simulink model "BatteryCCCV"  (R2023b)
settings: Solver=VariableStepAuto  StartTime=0.0  StopTime=5*23*3600  FixedStep=Ts  RelTol=1e-3  EnableMultiTasking=on
PreLoadFcn:
  | BatteryCCCVData;
values from neighbouring files (symbols this model uses):
  Ki = 10    [PVSystem_data.m]    (also in Simulink_INPUT_DATA_modified.m)
  Kp = 100    [PVSystem_data.m]    (also in Simulink_INPUT_DATA_modified.m)
  sim_avg_effectiveness_factor = mean(effectiveness_factors)    [Simulink_INPUT_DATA_modified.m]
  sim_general_loss_factor = general_loss_factor    [Simulink_INPUT_DATA_modified.m]
  sim_soiling_loss_factor = soiling_loss_factor    [Simulink_INPUT_DATA_modified.m]
  Ts = 1    [PVSystem_data.m]    (also in Simulink_INPUT_DATA_modified.m)
libraries: nesl_utility x4, fl_lib x3, simulink x2, batteryecm_lib x1, BatteryCurrentManagement x1
CloseFcn:
  | try
  |     close(h1_BatteryCCCV)
  | catch
  | end
  | 
  | clear h1_BatteryCCCV
  | 
  | clear BatteryCCCVSimlog
  | clear BatteryCCCVLogsout
  | 
  | clear AH SOC_vec T_vec R0_mat R1_mat tau1_mat
  | clear V0_mat initialSOC Ts vMax Kp Ki Kaw
  | clear cell_area h_conv thermal_mass
Description:
  | Battery charging and discharging
settings Model: Creator=The MathWorks, Inc.  LastModifiedBy=z004p7rb
settings SolverCC: AlgebraicLoopSolver=TrustRegion  MaxZcPerStep=1
settings DataIOCC: MaxDataPoints=370000  ReturnWorkspaceOutputs=off  SignalLoggingName=BatteryCCCVLogsout
settings OptimizationCC: ReuseModelBlockBuffer=off  LifeSpan=inf
settings DebuggingCC: UnconnectedInputMsg=warning  UnconnectedOutputMsg=warning  UnconnectedLineMsg=warning  SFUnexpectedBacktrackingDiag=warning  SFNoUnconditionalDefaultTransitionDiag=warning  SFExecutionAtInitializationDiag=none  ArithmeticOperatorsInVariantConditions=warning
settings ModelReferenceCC: EnableRefExpFcnMdlSchedulingChecks=on
settings SFSimCC: SimUseLocalCustomCode=off  CustomCodeUndefinedFunction=UseInterfaceOnly
settings RTWCC: RTWUseLocalCustomCode=off  DLArmComputeVersion=19.05
settings CodeAppCC: StateflowObjectComments=on
settings GRTTargetCC: TargetLangStandard=C89/C90 (ANSI)
settings ConfigComp: CovMetricSettings=dw  CovSaveCumulativeToWorkspaceVar=on  CovSaveSingleToWorkspaceVar=on  CovExternalEMLEnable=off
settings SimscapeCC: SimscapeLogType=all  SimscapeLogSimulationStatistics=on  SimscapeLogName=BatteryCCCVSimlog  SimscapeLogLimitData=off  SimscapeLogDataHistory=370000

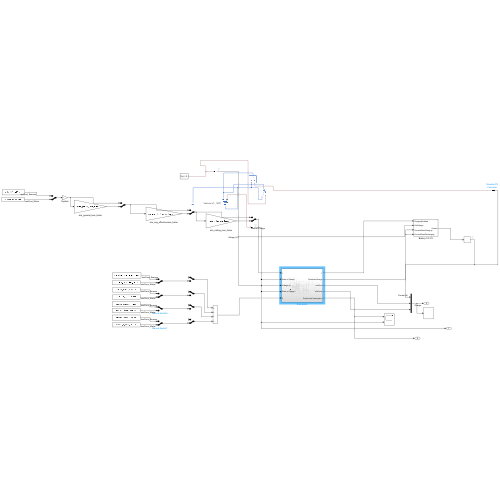
[thumbnail: Simulink's stored preview of the top-level diagram]
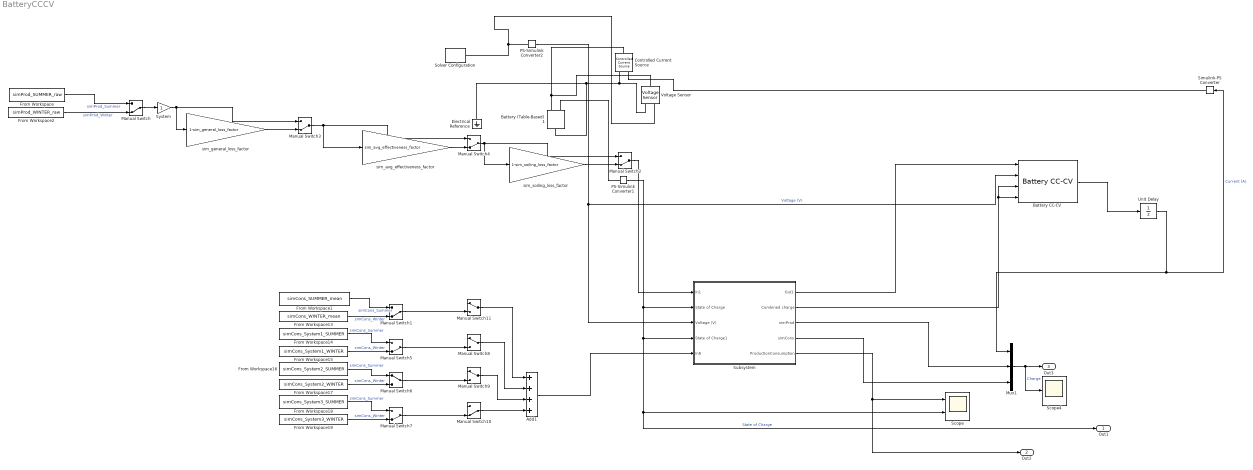
== system BatteryCCCV ==
  Add1 : Sum  Inputs=++++
  Battery (Table-Based)1 : batteryecm_lib/Battery (Table-Based)  Tag={'toolbox/physmod/battery/shared_library/m/batteryecm_lib_parts';'Battery__Table_Based_/Valence/U1_12XP.xml'}  SOC_vec=[0 0.01 0.02 0.03 0.04 0.05 0.06 0.07 0.08 0.09 0.1 0.11 0.12 0.13 0.14 0.15 0.16 0.17 0.18 0.19 0.2 0.21 0.22 0.23 0.24 0.25 0.26 0.27 0.28 0.29 0.3 0.31 0.32 0.33 0.34 0.35 0.36 0.37 0.38 0.39 0.4 0.41 0.42 0.43 0.44 0.45 0.46 0.47 0.48 0.49 0.5 0.51 0.52 0.53 0.54 0.55 0.56 0.57 0.58 0.59 0.6 0.61 0.62 0.63 0.64 0.65 0.66 0.67 0.68 0.69 0.7 0.71 0.72 0.73 0.74 0.75 0.76 0.77 0.78 0.79 0.8 0.81 0.82 0.83 0.84 0.85 0.86 0.87 0.88 0.89 0.9 0.91 0.92 0.93 0.94 0.95 0.96 0.97 0.98 0.99 1]  T_dependence=simscape.enum.tablebattery.temperature_dependence.no  prm_dir=simscape.enum.tablebattery.prm_dir.noCurrentDirectionality  T_vec=[-10 0 10 20 23 30 40] degC  V0_mat=[12.00518 12.00518 12.00518 12.00518 12.00518 12.00518 12.00518;12.046 12.046 12.046 12.046 12.046 12.046 12.046;12.08682 12.08682 12.08682 12.08682 12.08682 12.08682 12.08682;12.12763 12.12763 12.12763 12.12763 12.12763 12.12763 12.12763;12.16845 12.16845 12.16845 12.16845 12.16845 12.16845 12.16845;12.20927 12.20927 12.20927 12.20927 12.20927 12.20927 12.20927;12.25009 12.25009 12.25009 12.25009 12.25009 12.25009 12.25009;12.29091 12.29091 12.29091 12.29091 12.29091 12.29091 12.29091;12.33173 12.33173 12.33173 12.33173 12.33173 12.33173 12.33173;12.37255 12.37255 12.37255 12.37255 12.37255 12.37255 12.37255;12.41337 12.41337 12.41337 12.41337 12.41337 12.41337 12.41337;12.45419 12.45419 12.45419 12.45419 12.45419 12.45419 12.45419;12.49501 12.49501 12.49501 12.49501 12.49501 12.49501 12.49501;12.53583 12.53583 12.53583 12.53583 12.53583 12.53583 12.53583;12.56952 12.56952 12.56952 12.56952 12.56952 12.56952 12.56952;12.60149 12.60149 12.60149 12.60149 12.60149 12.60149 12.60149;12.63628 12.63628 12.63628 12.63628 12.63628 12.63628 12.63628;12.66676 12.66676 12.66676 12.66676 12.66676 12.66676 12.66676;12.6925 12.6925 12.6925 12.6925 12.6925 12.6925 12.6925;12.71984 12.71984 12.71984 12.71984 12.71984 12.71984 12.71984;12.74668 12.74668 12.74668 12.74668 12.74668 12.74668 12.74668;12.7709 12.7709 12.7709 12.7709 12.7709 12.7709 12.7709;12.79145 12.79145 12.79145 12.79145 12.79145 12.79145 12.79145;12.81167 12.81167 12.81167 12.81167 12.81167 12.81167 12.81167;12.82987 12.82987 12.82987 12.82987 12.82987 12.82987 12.82987;12.84554 12.84554 12.84554 12.84554 12.84554 12.84554 12.84554;12.85927 12.85927 12.85927 12.85927 12.85927 12.85927 12.85927;12.87336 12.87336 12.87336 12.87336 12.87336 12.87336 12.87336;12.8878 12.8878 12.8878 12.8878 12.8878 12.8878 12.8878;12.90226 12.90226 12.90226 12.90226 12.90226 12.90226 12.90226;12.91618 12.91618 12.91618 12.91618 12.91618 12.91618 12.91618;12.92892 12.92892 12.92892 12.92892 12.92892 12.92892 12.92892;12.9409 12.9409 12.9409 12.9409 12.9409 12.9409 12.9409;12.95179 12.95179 12.95179 12.95179 12.95179 12.95179 12.95179;12.96212 12.96212 12.96212 12.96212 12.96212 12.96212 12.96212;12.9718 12.9718 12.9718 12.9718 12.9718 12.9718 12.9718;12.98121 12.98121 12.98121 12.98121 12.98121 12.98121 12.98121;12.9894 12.9894 12.9894 12.9894 12.9894 12.9894 12.9894;12.99628 12.99628 12.99628 12.99628 12.99628 12.99628 12.99628;13.00194 13.00194 13.00194 13.00194 13.00194 13.00194 13.00194;13.00687 13.00687 13.00687 13.00687 13.00687 13.00687 13.00687;13.01127 13.01127 13.01127 13.01127 13.01127 13.01127 13.01127;13.01612 13.01612 13.01612 13.01612 13.01612 13.01612 13.01612;13.0201 13.0201 13.0201 13.0201 13.0201 13.0201 13.0201;13.0231 13.0231 13.0231 13.0231 13.0231 13.0231 13.0231;13.0261 13.0261 13.0261 13.0261 13.0261 13.0261 13.0261;13.02911 13.02911 13.02911 13.02911 13.02911 13.02911 13.02911;13.03211 13.03211 13.03211 13.03211 13.03211 13.03211 13.03211;13.03451 13.03451 13.03451 13.03451 13.03451 13.03451 13.03451;13.03664 13.03664 13.03664 13.03664 13.03664 13.03664 13.03664;13.03933 13.03933 13.03933 13.03933 13.03933 13.03933 13.03933;13.04232 13.04232 13.04232 13.04232 13.04232 13.04232 13.04232;13.04573 13.04573 13.04573 13.04573 13.04573 13.04573 13.04573;13.04919 13.04919 13.04919 13.04919 13.04919 13.04919 13.04919;13.05277 13.05277 13.05277 13.05277 13.05277 13.05277 13.05277;13.05642 13.05642 13.05642 13.05642 13.05642 13.05642 13.05642;13.06013 13.06013 13.06013 13.06013 13.06013 13.06013 13.06013;13.06395 13.06395 13.06395 13.06395 13.06395 13.06395 13.06395;13.06828 13.06828 13.06828 13.06828 13.06828 13.06828 13.06828;13.07261 13.07261 13.07261 13.07261 13.07261 13.07261 13.07261;13.07686 13.07686 13.07686 13.07686 13.07686 13.07686 13.07686;13.08121 13.08121 13.08121 13.08121 13.08121 13.08121 13.08121;13.08594 13.08594 13.08594 13.08594 13.08594 13.08594 13.08594;13.09142 13.09142 13.09142 13.09142 13.09142 13.09142 13.09142;13.09708 13.09708 13.09708 13.09708 ...(+2253 chars)] V  V0_vec=[12.00518 12.046 12.08682 12.12763 12.16845 12.20927 12.25009 12.29091 12.33173 12.37255 12.41337 12.45419 12.49501 12.53583 12.56952 12.60149 12.63628 12.66676 12.6925 12.71984 12.74668 12.7709 12.79145 12.81167 12.82987 12.84554 12.85927 12.87336 12.8878 12.90226 12.91618 12.92892 12.9409 12.95179 12.96212 12.9718 12.98121 12.9894 12.99628 13.00194 13.00687 13.01127 13.01612 13.0201 13.0231 13.0261 13.02911 13.03211 13.03451 13.03664 13.03933 13.04232 13.04573 13.04919 13.05277 13.05642 13.06013 13.06395 13.06828 13.07261 13.07686 13.08121 13.08594 13.09142 13.09708 13.10279 13.10857 13.11438 13.12019 13.1263 13.13263 13.13899 13.14595 13.15268 13.15967 13.16669 13.17384 13.17943 13.18402 13.18838 13.19255 13.19694 13.20123 13.20527 13.20912 13.2115 13.21389 13.21588 13.21758 13.21949 13.22126 13.224 13.227 13.23066 13.23444 13.23732 13.23875 13.23911 13.23888 13.25149 13.31471] V  V_range=[12.00518 13.31471] V  R0_mat=[0.31149 0.24646 0.1305 0.14557 0.06981 0.12094 0.10043;0.31245 0.23652 0.11852 0.12502 0.0625 0.09416 0.06761;0.30299 0.22658 0.10654 0.10446 0.05518 0.071 0.05004;0.29352 0.21664 0.09456 0.08497 0.04785 0.05545 0.03565;0.28405 0.2067 0.08326 0.0695 0.04083 0.04376 0.02394;0.27458 0.19676 0.07425 0.05748 0.03437 0.03259 0.01541;0.26512 0.18683 0.06508 0.0482 0.02911 0.02462 0.00923;0.25565 0.17689 0.05699 0.04095 0.02515 0.01945 0.00517;0.24618 0.16695 0.05025 0.03428 0.02195 0.01534 0.00236;0.23671 0.15701 0.04492 0.02949 0.01956 0.0115 0.00085;0.22724 0.14707 0.04118 0.02542 0.01764 0.00986 0.00061;0.21778 0.13713 0.03744 0.02233 0.01618 0.00823 0.00064;0.20831 0.12719 0.03369 0.01978 0.01518 0.00787 0.00119;0.19884 0.11725 0.03108 0.01847 0.01436 0.00758 0.00174;0.18937 0.10701 0.0287 0.01681 0.01349 0.00698 0.00186;0.1799 0.09743 0.02624 0.01521 0.01311 0.00656 0.00189;0.17044 0.08843 0.02418 0.01493 0.01277 0.00629 0.00207;0.16097 0.08111 0.0236 0.01443 0.01245 0.00644 0.00225;0.1515 0.074 0.02279 0.01369 0.01206 0.00666 0.00245;0.14203 0.0677 0.02206 0.01303 0.01189 0.00696 0.00273;0.13257 0.06168 0.0213 0.01283 0.01179 0.00725 0.00299;0.12217 0.05582 0.02087 0.01288 0.01168 0.00749 0.00323;0.11213 0.0525 0.02085 0.01275 0.01153 0.00754 0.00344;0.10314 0.04948 0.02082 0.0126 0.01152 0.00757 0.00364;0.09444 0.04636 0.02069 0.01235 0.01151 0.0075 0.00376;0.08561 0.04418 0.02043 0.01214 0.01146 0.00748 0.0039;0.07908 0.04215 0.02007 0.01218 0.0114 0.00741 0.00395;0.073 0.04014 0.01973 0.01225 0.01137 0.00737 0.00401;0.06878 0.03834 0.01964 0.01233 0.01137 0.00734 0.00403;0.06496 0.03708 0.01958 0.01241 0.01138 0.00731 0.00405;0.06117 0.0358 0.01949 0.01246 0.0114 0.00726 0.00405;0.05837 0.03446 0.01935 0.01262 0.01143 0.00716 0.00415;0.05554 0.0331 0.01917 0.01274 0.01146 0.00743 0.00426;0.05334 0.0326 0.01893 0.01281 0.01148 0.00765 0.00437;0.05171 0.03208 0.01888 0.01285 0.01149 0.00784 0.00451;0.05005 0.03152 0.01897 0.01286 0.0115 0.00799 0.00462;0.04837 0.03123 0.01906 0.01285 0.01151 0.00813 0.00474;0.04707 0.03089 0.01908 0.01288 0.01153 0.00821 0.00481;0.04632 0.03049 0.01903 0.01286 0.01152 0.00823 0.00482;0.04552 0.03007 0.01892 0.01278 0.0115 0.00818 0.00477;0.04468 0.02982 0.01878 0.01267 0.01147 0.00814 0.00471;0.04381 0.02954 0.01861 0.01253 0.01143 0.00809 0.00463;0.04296 0.02929 0.01847 0.01241 0.01141 0.00807 0.00457;0.04221 0.02899 0.0184 0.01224 0.01138 0.008 0.00447;0.04182 0.02866 0.01828 0.01203 0.01134 0.00789 0.00432;0.04143 0.02837 0.01816 0.01182 0.0113 0.00777 0.00417;0.04103 0.02807 0.01804 0.01172 0.01126 0.00767 0.00402;0.04064 0.02778 0.01792 0.01163 0.01122 0.00757 0.00401;0.04022 0.02746 0.01777 0.0115 0.01117 0.00745 0.00397;0.03979 0.02712 0.0176 0.01136 0.01113 0.00731 0.00391;0.03964 0.02688 0.01747 0.01125 0.0111 0.0072 0.00389;0.03949 0.02672 0.01735 0.01116 0.01108 0.0071 0.00387;0.03937 0.02658 0.01725 0.01108 0.01106 0.00705 0.00387;0.03925 0.02644 0.01717 0.01101 0.01105 0.00699 0.00387;0.03914 0.02631 0.01711 0.01094 0.01104 0.00695 0.00385;0.03903 0.02618 0.01705 0.01092 0.01103 0.0069 0.00384;0.03892 0.0262 0.017 0.01089 0.01102 0.00686 0.00382;0.03882 0.02624 0.01695 0.01087 0.01101 0.00683 0.00382;0.03877 0.02629 0.01693 0.01088 0.01102 0.00683 0.00387;0.0389 0.02635 0.01691 0.01089 0.01104 0.00684 0.00391;0.03901 0.0264 0.01689 0.01089 0.01105 0.00685 0.00396;0.03914 0.02644 0.01687 0.0109 0.01107 0.00686 0.004;0.03928 0.02648 0.01687 0.01093 0.01109 0.00689 0.00407;0.03946 0.02656 0.01694 0.011 0.01113 0.00695 0.00415;0.03965 0.02665 0.01709 0.01108 0.01117 0.00703 0.00425;0.03995 0.02674 0.01724 0.01117 0.01122 0.00714 0.00434;0.04035 0.02683 0.01739 0.01126 0.01127 0.00725 0.00443;0.04075 0.02692 0.01754 0.01136 0.01131 0.00736 0.00452;0.04115 0.02711 0.0177 0.01145 0.01136 0.00747 0.00461;0.04157 0.02734 0.01787 0.01156 0.01142 0.00759 0.00472;0.04196 0.02759 0.01803 0.01168 0.01148 0.00773 0.00483;0.04232 0.02783 0.01813 0.01181 0.01153 0.00786 0.00495;0.04271 0.02811 ...(+1584 chars)] Ohm  R0_vec=[0.06981 0.0625 0.05518 0.04785 0.04083 0.03437 0.02911 0.02515 0.02195 0.01956 0.01764 0.01618 0.01518 0.01436 0.01349 0.01311 0.01277 0.01245 0.01206 0.01189 0.01179 0.01168 0.01153 0.01152 0.01151 0.01146 0.0114 0.01137 0.01137 0.01138 0.0114 0.01143 0.01146 0.01148 0.01149 0.0115 0.01151 0.01153 0.01152 0.0115 0.01147 0.01143 0.01141 0.01138 0.01134 0.0113 0.01126 0.01122 0.01117 0.01113 0.0111 0.01108 0.01106 0.01105 0.01104 0.01103 0.01102 0.01101 0.01102 0.01104 0.01105 0.01107 0.01109 0.01113 0.01117 0.01122 0.01127 0.01131 0.01136 0.01142 0.01148 0.01153 0.0116 0.01166 0.01174 0.01182 0.0119 0.01195 0.012 0.01204 0.01209 0.01214 0.01219 0.01223 0.01227 0.01226 0.01225 0.01223 0.01221 0.01217 0.01212 0.01208 0.01205 0.01201 0.01196 0.01184 0.0117 0.01136 0.01069 0.0098 0.00774] Ohm  R0_dis_mat=[.0117, .0085, .009; .011, .0085, .009; .0114, .0087, .0092; .0107, .0082, .0088; .0107, .0083, .0091; .0113, .0085, .0089; .0116, .0085, .0089] % Parameter not set Ohm  R0_dis_vec=[.0085, .0085, .0087, .0082, .0083, .0085, .0085] % Parameter not set Ohm  R0_ch_mat=[.0117, .0085, .009; .011, .0085, .009; .0114, .0087, .0092; .0107, .0082, .0088; .0107, .0083, .0091; .0113, .0085, .0089; .0116, .0085, .0089] % Parameter not set Ohm  R0_ch_vec=[.0085, .0085, .0087, .0082, .0083, .0085, .0085] % Parameter not set Ohm  AH=AH_system1 hr*A  prm_leak=simscape.enum.tablebattery.prm_leak.disabled  Rleak_vec=[8000, 7000, 6000] % Parameter not set Ohm  Rleak=7e3 % Parameter not set Ohm  extrapolation_option=simscape.enum.extrapolation.nearest  SOC_port=simscape.enum.tablebattery.enable.yes  prm_dyn=simscape.enum.tablebattery.prm_dyn.off  R1_mat=[.0109, .0029, .0013; .0069, .0024, .0012; .0047, .0026, .0013; .0034, .0016, .001; .0033, .0023, .0014; .0033, .0018, .0011; .0028, .0017, .0011] % Parameter not set Ohm  R1_vec=[.0029, .0024, .0026, .0016, .0023, .0018, .0017] % Parameter not set Ohm  tau1_mat=[20, 36, 39; 31, 45, 39; 109, 105, 61; 36, 29, 26; 59, 77, 67; 40, 33, 29; 25, 39, 33] % Parameter not set s  tau1_vec=[36, 45, 105, 29, 77, 33, 39] % Parameter not set s  R2_mat=[.0109, .0029, .0013; .0069, .0024, .0012; .0047, .0026, .0013; .0034, .0016, .001; .0033, .0023, .0014; .0033, .0018, .0011; .0028, .0017, .0011] % Parameter not set Ohm  R2_vec=[.0029, .0024, .0026, .0016, .0023, .0018, .0017] % Parameter not set Ohm  tau2_mat=[20, 36, 39; 31, 45, 39; 109, 105, 61; 36, 29, 26; 59, 77, 67; 40, 33, 29; 25, 39, 33] % Parameter not set s  tau2_vec=[36, 45, 105, 29, 77, 33, 39] % Parameter not set s  R3_mat=[.0109, .0029, .0013; .0069, .0024, .0012; .0047, .0026, .0013; .0034, .0016, .001; .0033, .0023, .0014; .0033, .0018, .0011; .0028, .0017, .0011] % Parameter not set Ohm  R3_vec=[.0029, .0024, .0026, .0016, .0023, .0018, .0017] % Parameter not set Ohm  tau3_mat=[20, 36, 39; 31, 45, 39; 109, 105, 61; 36, 29, 26; 59, 77, 67; 40, 33, 29; 25, 39, 33] % Parameter not set s  tau3_vec=[36, 45, 105, 29, 77, 33, 39] % Parameter not set s  R4_mat=[.0109, .0029, .0013; .0069, .0024, .0012; .0047, .0026, .0013; .0034, .0016, .001; .0033, .0023, .0014; .0033, .0018, .0011; .0028, .0017, .0011] % Parameter not set Ohm  R4_vec=[.0029, .0024, .0026, .0016, .0023, .0018, .0017] % Parameter not set Ohm  tau4_mat=[20, 36, 39; 31, 45, 39; 109, 105, 61; 36, 29, 26; 59, 77, 67; 40, 33, 29; 25, 39, 33] % Parameter not set s  tau4_vec=[36, 45, 105, 29, 77, 33, 39] % Parameter not set s  R5_mat=[.0109, .0029, .0013; .0069, .0024, .0012; .0047, .0026, .0013; .0034, .0016, .001; .0033, .0023, .0014; .0033, .0018, .0011; .0028, .0017, .0011] % Parameter not set Ohm  R5_vec=[.0029, .0024, .0026, .0016, .0023, .0018, .0017] % Parameter not set Ohm  tau5_mat=[20, 36, 39; 31, 45, 39; 109, 105, 61; 36, 29, 26; 59, 77, 67; 40, 33, 29; 25, 39, 33] % Parameter not set s  tau5_vec=[36, 45, 105, 29, 77, 33, 39] % Parameter not set s  prm_fade=simscape.enum.tablebattery.prm_fade.tableN  N0=100 % Parameter not set  dV0=0 % Parameter not set  dR0=0 % Parameter not set  dAH=0 % Parameter not set  dRleak=0 % Parameter not set  dR1=0 % Parameter not set  dR2=0 % Parameter not set  dR3=0 % Parameter not set  dR4=0 % Parameter not set  dR5=0 % Parameter not set  N0vec=[0 49 97 145 193 241 289 337 385 433 481 529 577 625 673 721 769 817 865 913 961 1009 1057 1105 1153 1201 1249 1297 1345 1393 1441 1489 1537 1585 1633 1681 1729 1777 1825 1873 1921 1969 2017 2065 2113 2161 2209 2257 2305 2353 2401 2449 2497 2545 2593 2641 2689 2737 2785 2833 2881 2929 2977 3025 3073 3121 3169 3217 3265 3313 3361 3409 3457 3505 3553 3601 3649 3697 3745 3793 3841 3889 3937 3985 4033 4081 4129 4177 4225 4273 4321 4369 4417 4465 4513 4561 4609 4657 4705 4753]  Tfadevec=[298.15, 323.15] % Parameter not set K  dV0vec=[0 -0.2242 -0.4483 -0.5142 -0.5589 -0.569 -0.5683 -0.5681 -0.5692 -0.5703 -0.5741 -0.5782 -0.5834 -0.5917 -0.6 -0.6099 -0.6207 -0.6305 -0.6399 -0.6492 -0.6586 -0.6663 -0.6741 -0.6817 -0.6907 -0.7003 -0.707 -0.7132 -0.7197 -0.7264 -0.7327 -0.7387 -0.7438 -0.7496 -0.7554 -0.7619 -0.7688 -0.7757 -0.7826 -0.7901 -0.8006 -0.813 -0.8255 -0.8384 -0.8519 -0.8664 -0.881 -0.8958 -0.9106 -0.9251 -0.9392 -0.9546 -0.972 -0.9899 -1.0083 -1.029 -1.0514 -1.0782 -1.1068 -1.135 -1.1599 -1.1836 -1.2073 -1.2304 -1.2531 -1.2762 -1.2997 -1.323 -1.3445 -1.366 -1.3874 -1.4088 -1.4297 -1.4544 -1.4788 -1.5029 -1.5269 -1.5509 -1.5749 -1.5987 -1.6223 -1.6459 -1.6686 -1.6899 -1.711 -1.7302 -1.7484 -1.7656 -1.7823 -1.7987 -1.8151 -1.8379 -1.8631 -1.8878 -1.9102 -1.9319 -1.9533 -1.9745 -1.9953 -2.0155]  dR0vec=[0 0 0 0 0 0 0 0 0 0 0 0 0 0 0 0 0 0 0 0 0 0 0 0 0 0 0 0 0 0 0 0 0 0 0 0 0 0 0 0 0 0 0 0 0 0 0 0 0 0 0 0 0 0 0 0 0 0 0 0 0 0 0 0 0 0 0 0 0 0 0 0 0 0 0 0 0 0 0 0 0 0 0 0 0 0 0 0 0 0 0 0 0 0 0 0 0 0 0 0] % Parameter assumed  dAHvec=[0 -0.472 -0.944 -1.416 -1.889 -2.306 -2.716 -3.125 -3.535 -3.944 -4.342 -4.723 -5.104 -5.485 -5.867 -6.248 -6.629 -6.972 -7.314 -7.656 -7.997 -8.339 -8.681 -9.022 -9.457 -9.923 -10.389 -10.855 -11.321 -11.787 -12.254 -12.72 -13.106 -13.491 -13.876 -14.262 -14.647 -15.032 -15.417 -15.837 -16.264 -16.69 -17.116 -17.542 -17.987 -18.438 -18.889 -19.341 -19.792 -20.243 -20.694 -21.177 -21.71 -22.243 -22.776 -23.309 -23.842 -24.376 -24.909 -25.442 -25.915 -26.366 -26.816 -27.266 -27.717 -28.167 -28.617 -29.068 -29.518 -29.968 -30.419 -30.869 -31.319 -31.858 -32.41 -32.961 -33.512 -34.063 -34.615 -35.166 -35.717 -36.269 -36.802 -37.314 -37.826 -38.339 -38.851 -39.363 -39.875 -40.388 -40.9 -41.603 -42.38 -43.158 -43.935 -44.712 -45.49 -46.267 -47.044 -47.822]  dRleakvec=[0, 0, 0] % Parameter not set  dR1vec=[0, 0, 0] % Parameter not set  dR2vec=[0, 0, 0] % Parameter not set  dR3vec=[0, 0, 0] % Parameter not set  dR4vec=[0, 0, 0] % Parameter not set  dR5vec=[0, 0, 0] % Parameter not set  dV0mat=[0, 0; 0, 0; 0, 0] % Parameter not set  dR0mat=[0, 0; 0, 0; 0, 0] % Parameter not set  dAHmat=[0, 0; 0, 0; 0, 0] % Parameter not set  dRleakmat=[0, 0; 0, 0; 0, 0] % Parameter not set  dR1mat=[0, 0; 0, 0; 0, 0] % Parameter not set  dR2mat=[0, 0; 0, 0; 0, 0] % Parameter not set  dR3mat=[0, 0; 0, 0; 0, 0] % Parameter not set  dR4mat=[0, 0; 0, 0; 0, 0] % Parameter not set  dR5mat=[0, 0; 0, 0; 0, 0] % Parameter not set  prm_age_modeling=simscape.enum.tablebattery.prm_age_modeling.equation  storage_dt_age_vec=[0] % Parameter not set d  storage_T_age_vec=[273] % Parameter not set K  prm_age_OCV=simscape.enum.tablebattery.prm_age_OCV.OCV  OCV_age=0.9 % Parameter not set  SOC_age=0.6 % Parameter not set  prm_age_resistance=simscape.enum.tablebattery.prm_age.disabled  OCV_scaling_age_resistance=2.2134e6 % Parameter not set  OCV_offset_age_resistance=1.632e6 % Parameter not set  temp_exp_age_resistance=0.515833569 % Parameter not set V  t_exp_age_resistance=0.75 % Parameter not set  T_age_vec_resistance=[273.15, 298.15, 323.15] % Parameter not set K  dt_age_vec_resistance=[90, 180, 270, 360] % Parameter not set d  dR0_age_vec=[0, 0, 0] % Parameter not set  t_meas_dR0_age=100 % Parameter not set d  dR0_age_mat=[0, 0, 0; 0, 0, 0; 0, 0, 0; 0, 0, 0] % Parameter not set  prm_age_capacity=simscape.enum.tablebattery.prm_age.disabled  OCV_scaling_age_capacity=1.5097e07 % Parameter not set  OCV_offset_age_capacity=8.3625e06 % Parameter not set  temp_exp_age_capacity=0.6011 % Parameter not set V  t_exp_age_capacity=0.75 % Parameter not set  T_age_vec_capacity=[273.15, 298.15, 323.15] % Parameter not set K  dt_age_vec_capacity=[90, 180, 270, 360] % Parameter not set d  dAH_age_vec=[0, 0, 0] % Parameter not set  t_meas_dAH_age=100 % Parameter not set d  dAH_age_mat=[0, 0, 0; 0, 0, 0; 0, 0, 0; 0, 0, 0] % Parameter not set  thermal_port=simscape.enum.thermaleffects.omit  temperature=298.15 % Parameter not set K  thermal_mass=5868 % Parameter assumed J/K  i_specify=off  i_priority=None  i=0 A  i_nominal_specify=off  i_nominal_unit=A  i_nominal_value=1  v_specify=off  v_priority=None  v=0 V  v_nominal_specify=off  v_nominal_unit=V  v_nominal_value=1  stateOfCharge_specify=on  stateOfCharge_priority=High  stateOfCharge=initialSOC  stateOfCharge_nominal_specify=off  stateOfCharge_nominal_unit=1  stateOfCharge_nominal_value=1  num_cycles_specify=off  num_cycles_priority=High  num_cycles=0  num_cycles_nominal_specify=off  num_cycles_nominal_unit=1  num_cycles_nominal_value=1  cell_temperature_specify=off  cell_temperature_priority=High  cell_temperature=298.15 K  cell_temperature_nominal_specify=off  cell_temperature_nominal_unit=K  cell_temperature_nominal_value=1
      settings: AttributesFormatString=Valence:U1_12XP  InternalSimscapePortConfiguration="{\"Bottom\":[],\"Left\":[{\"id\":\"p\",\"label\":\"+\",\"type\":\"foundation.electrical.electrical\"},{\"id\":\"soc\",\"label\":\"SOC\",\"type\":\"output\"}],\"Right\":[{\"id\":\"n\",\"label\":\"-\",\"type\":\"foundation.electrical.electrical\"}],\"Top\":[]}"
      settings: LibrarySourceBlock=|
      | batt_lib/Cells/Battery
      | (Table-Based)
  Battery CC-CV : BatteryCurrentManagement/Battery CC-CV  MaxCellVoltage=13.31471  Kp=Kp  Ki=Ki  Kaw=Kaw  Kt=1  Ts=Ts
      settings: LibrarySourceBlock=batt_sl_lib/Current Management/Battery CC-CV
  Controlled Current Source : fl_lib/Electrical/Electrical Sources/Controlled Current Source
  Electrical Reference : fl_lib/Electrical/Electrical Elements/Electrical Reference
  From Workspace : FromWorkspace  VariableName=simProd_SUMMER_raw
  From Workspace1 : FromWorkspace  VariableName=simCons_SUMMER_mean
  From Workspace13 : FromWorkspace  VariableName=simCons_WINTER_mean
  From Workspace14 : FromWorkspace  VariableName=simCons_System1_SUMMER
  From Workspace15 : FromWorkspace  VariableName=simCons_System1_WINTER
  From Workspace16 : FromWorkspace  VariableName=simCons_System2_SUMMER
  From Workspace17 : FromWorkspace  VariableName=simCons_System2_WINTER
  From Workspace18 : FromWorkspace  VariableName=simCons_System3_SUMMER
  From Workspace19 : FromWorkspace  VariableName=simCons_System3_WINTER
  From Workspace2 : FromWorkspace  VariableName=simProd_WINTER_raw
  Manual Switch{,1..5,7,10} (8 alike) : ManualSwitch  CurrentSetting=0
  Manual Switch{6,8..9,11} (4 alike) : ManualSwitch
  Mux1 : Mux  Inputs=3
  PS-Simulink Converter1 : nesl_utility/PS-Simulink Converter  PhysicalDomain=network_engine_domain  SubClassName=ps_output  LeftPortType=input  RightPortType=output  PseudoPeriodic=off  Frequencies=[]  VectorFormat=inherit  Unit=inherit  AffineConversion=off
  PS-Simulink Converter2 : nesl_utility/PS-Simulink Converter  PhysicalDomain=network_engine_domain  SubClassName=ps_output  LeftPortType=input  RightPortType=output  PseudoPeriodic=off  Frequencies=[]  VectorFormat=inherit  Unit=inherit  AffineConversion=off
  Scope : Scope  NumInputPorts=2
  Scope4 : Scope
  Simulink-PS Converter : nesl_utility/Simulink-PS Converter  PhysicalDomain=network_engine_domain  SubClassName=ps_input  LeftPortType=input  RightPortType=output  PseudoPeriodic=off  Frequencies=[]  NoiseDistribution=none  NoiseParameters=[]  Unit=1  AffineConversion=off  FilteringAndDerivatives=provide  SimscapeFilterOrder=1  InputFilterTimeConstant=0.001  UdotUserProvided=0
  Solver Configuration : nesl_utility/Solver Configuration  PhysicalDomain=network_engine_domain  SubClassName=solver  LeftPortType=input  RightPortType=generic  Tones=[]  Harmonics=[]  SimulateNoise=off  Profile=off  UseLocalSampling=off  EnableSwitchedLinearOptims=on  FrequencyDomain=off  UseCCode=off  RelTol=0.001  AbsTol=0.001  MinStep=1e-09  ToWorkspace=off  RevertToSquareIcSolve=off  NumHomotopyIterations=100  PhasorMode=off  PhasorModeNumHarmonics=1  ConsistencySolver=NEWTON_XTOL_AFTER_FTOL  IndexReductionMethod=DerivativeReplacement  DoDC=off  ResidualTolerance=1e-09  ConsistencyTolSource=GLOBAL  ConsistencyAbsTol=0.001  ConsistencyRelTol=0.001  ConsistencyTolFactor=0.001  UseLocalSolver=off  LocalSolverChoice=NE_BACKWARD_EULER_ADVANCER  ResolveIndetEquations=on  FunctionEvalNumThread=1  LocalSolverSampleTime=0.001  DoFixedCost=off  MaxNonlinIter=3  MaxModeIter=2  ComputeImpulses=off  ImpulseIterations=2  LinearAlgebra=auto  LinearAlgebraNumThread=0  EquationFormulation=NE_TIME_EF  DelaysMemoryBudget=1024  AutomaticFiltering=on  FilteringTimeConstant=0.001  PartitionStorageMethod=AS_NEEDED  PartitionMemoryBudget=1024  PartitionMethod=ROBUST  MultibodyUseLocalSolver=off  MultibodyLocalSolverChoice=ODE1  MultibodyLocalSolverSampleTime=0.001
  Subsystem : Subsystem
  System : Gain
  Unit Delay : UnitDelay  SampleTime=-1  HasFrameUpgradeWarning=on
  Voltage Sensor : fl_lib/Electrical/Electrical Sensors/Voltage Sensor
  sim_avg_effectiveness_factor : Gain  Gain=sim_avg_effectiveness_factor
  sim_general_loss_factor : Gain  Gain=1-sim_general_loss_factor
  sim_soiling_loss_factor : Gain  Gain=1-sim_soiling_loss_factor
  Out1 : Outport
  Out2 : Outport  Port=2
  Out3 : Outport  Port=3
  wires:
  From Workspace1/1 -> Manual Switch1/1  "simCons_Summer"
  From Workspace/1 -> Manual Switch/1  "simProd_Summer"
  Manual Switch10/1 -> Add1/4
  From Workspace2/1 -> Manual Switch/2  "simProd_Winter"
  PS-Simulink Converter1/1 -> Subsystem/2(State of Charge), Scope/2, Out1/1, Subsystem/4(State of Charge1)  "State of Charge"
  Manual Switch/1 -> System/1
  Manual Switch8/1 -> Add1/2
  System/1 -> Manual Switch3/1, sim_general_loss_factor/1
  sim_general_loss_factor/1 -> Manual Switch3/2
  Manual Switch3/1 -> Manual Switch4/1, sim_avg_effectiveness_factor/1
  From Workspace13/1 -> Manual Switch1/2  "simCons_Winter"
  From Workspace17/1 -> Manual Switch6/2  "simCons_Winter"
  From Workspace14/1 -> Manual Switch5/1  "simCons_Summer"
  From Workspace15/1 -> Manual Switch5/2  "simCons_Winter"
  From Workspace16/1 -> Manual Switch6/1  "simCons_Summer"
  From Workspace18/1 -> Manual Switch7/1  "simCons_Summer"
  From Workspace19/1 -> Manual Switch7/2  "simCons_Winter"
  sim_avg_effectiveness_factor/1 -> Manual Switch4/2
  Manual Switch1/1 -> Manual Switch11/2
  Manual Switch5/1 -> Manual Switch8/2
  Manual Switch6/1 -> Manual Switch9/2
  Manual Switch9/1 -> Add1/3
  Manual Switch7/1 -> Manual Switch10/2
  Manual Switch4/1 -> Manual Switch2/1, sim_soiling_loss_factor/1
  Manual Switch11/1 -> Add1/1
  sim_soiling_loss_factor/1 -> Manual Switch2/2
  PS-Simulink Converter2/1 -> Subsystem/3(Voltage (V)), Battery CC-CV/2  "Voltage (V)"
  Battery CC-CV/1 -> Unit Delay/1
  Unit Delay/1 -> Mux1/1, Simulink-PS Converter/1  "Current (A)"
  Mux1/1 -> Out3/1, Scope4/1  "Charge"
  Subsystem/5(ProductionConsumption) -> Scope/1, Out2/1
  Subsystem/2(Combined charge) -> Battery CC-CV/3, Battery CC-CV/4
  Manual Switch2/1 -> Subsystem/1(In1)
  Add1/1 -> Subsystem/5(In8)
  Subsystem/1(Out1) -> Battery CC-CV/1
  Subsystem/3(simProd) -> Mux1/2
  Subsystem/4(simCons) -> Mux1/3
  connections:
  Electrical Reference/LConn1 -- Controlled Current Source/RConn2 -- Voltage Sensor/RConn2 -- Battery (Table-Based)1/RConn1
  PS-Simulink Converter2/LConn1 -- Solver Configuration/RConn1 -- Voltage Sensor/RConn1
  Battery (Table-Based)1/LConn1 -- Controlled Current Source/LConn1 -- Voltage Sensor/LConn1
  Battery (Table-Based)1/LConn2 -- PS-Simulink Converter1/LConn1
  Controlled Current Source/RConn1 -- Simulink-PS Converter/RConn1

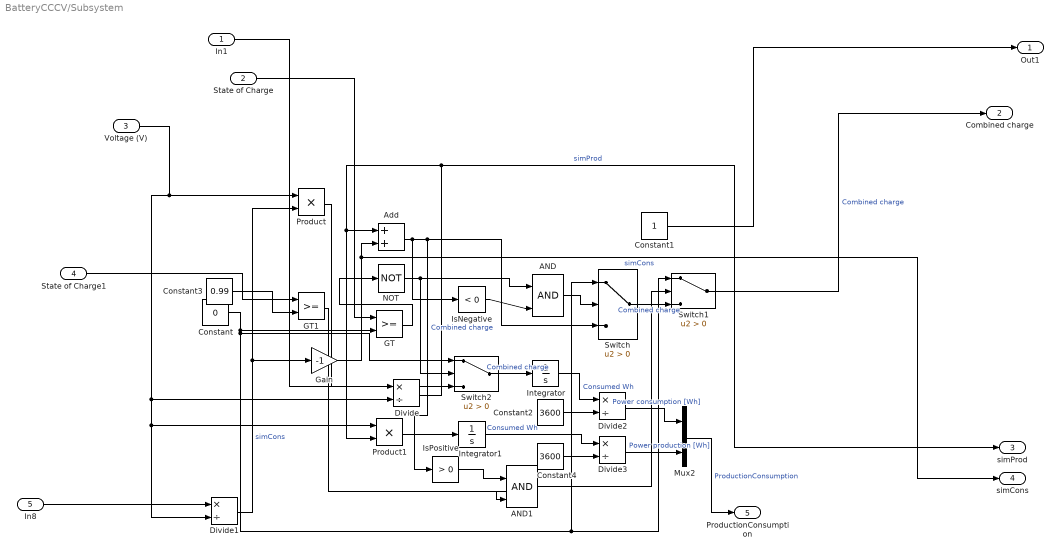
== system BatteryCCCV/Subsystem ==
  In1 : Inport
  State of Charge : Inport  Port=2
  Voltage (V) : Inport  Port=3
  State of Charge1 : Inport  Port=4
  In8 : Inport  Port=5
  AND : Logic  IconShape=distinctive  AllPortsSameDT=off  OutDataTypeStr=boolean
  AND1 : Logic  IconShape=distinctive  AllPortsSameDT=off  OutDataTypeStr=boolean
  Add : Sum
  Constant : Constant  Value=0
  Constant1 : Constant
  Constant2 : Constant  Value=3600
  Constant3 : Constant  Value=0.99
  Constant4 : Constant  Value=3600
  Divide{,1..3} (4 alike) : Product  Inputs=*/
  GT : RelationalOperator  OutDataTypeStr=boolean  RndMeth=Simplest  InputSameDT=off
  GT1 : RelationalOperator  OutDataTypeStr=boolean  RndMeth=Simplest  InputSameDT=off
  Gain : Gain  Gain=-1
  Integrator : Integrator
  Integrator1 : Integrator
  IsNegative : simulink/Logic and Bit Operations/Compare To Zero  relop=<  OutDataTypeStr=boolean
      settings: LibrarySourceBlock=|
      | simulink/Quick Insert/Logic and Bit
      | Operations/IsNegative
  IsPositive : simulink/Logic and Bit Operations/Compare To Zero  relop=>  OutDataTypeStr=boolean
      settings: LibrarySourceBlock=|
      | simulink/Quick Insert/Logic and Bit
      | Operations/IsPositive
  Mux2 : Mux  Inputs=2
  NOT : Logic  Operator=NOT  IconShape=distinctive  AllPortsSameDT=off  OutDataTypeStr=boolean
  Product : Product
  Product1 : Product
  Switch : Switch  Criteria=u2 > Threshold  SaturateOnIntegerOverflow=off  InputSameDT=off
  Switch1 : Switch  Criteria=u2 > Threshold  SaturateOnIntegerOverflow=off  InputSameDT=off
  Switch2 : Switch  Criteria=u2 > Threshold  SaturateOnIntegerOverflow=off  InputSameDT=off
  Out1 : Outport
  Combined charge : Outport  Port=2
  simProd : Outport  Port=3
  simCons : Outport  Port=4
  ProductionConsumption : Outport  Port=5
  wires:
  GT1/1 -> AND1/2
  Divide1/1 -> Product/2, Gain/1  "simCons"
  AND1/1 -> Switch1/2
  Switch2/1 -> Integrator/1  "Combined charge"
  Voltage (V)/1 -> Divide/2, Product1/1, Divide1/2, Product/1
  AND/1 -> Switch/2
  Add/1 -> Switch/3, IsPositive/1, IsNegative/1  "Combined charge"
  Gain/1 -> Add/2, simCons/1  "simCons"
  IsNegative/1 -> AND/2
  Constant/1 -> Switch1/1, Switch/1, Switch2/1, GT/2
  Divide2/1 -> Mux2/1  "Power consumption [Wh]"
  Constant2/1 -> Divide2/2
  Product/1 -> Switch2/3
  GT/1 -> NOT/1
  Constant3/1 -> GT1/2
  Product1/1 -> Integrator1/1
  State of Charge1/1 -> GT1/1
  Constant4/1 -> Divide3/2
  Integrator/1 -> Divide2/1  "Consumed Wh"
  Mux2/1 -> ProductionConsumption/1  "ProductionConsumption"
  IsPositive/1 -> AND1/1
  State of Charge/1 -> GT/1
  Integrator1/1 -> Divide3/1  "Consumed Wh"
  NOT/1 -> AND/1, Switch2/2
  In8/1 -> Divide1/1
  Divide/1 -> simProd/1, Add/1, Product1/2  "simProd"
  Switch/1 -> Switch1/3  "Combined charge"
  Divide3/1 -> Mux2/2  "Power production [Wh]"
  Switch1/1 -> Combined charge/1  "Combined charge"
  In1/1 -> Divide/1
  Constant1/1 -> Out1/1
